simulink model "LimKyuBum_20101447_5"  (R2017a)
settings: Solver=VariableStepAuto  StartTime=0.0  StopTime=10.0  RelTol=1e-3
settings Model: Creator=508-104  LastModifiedBy=508-104

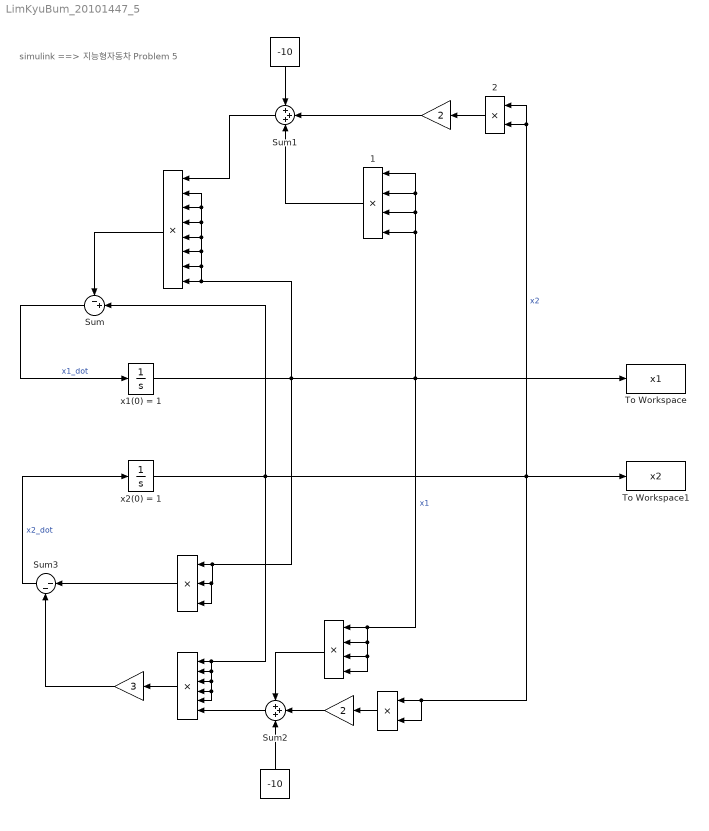
== system LimKyuBum_20101447_5 ==
  note: simulink ==> 지능형자동차 Problem 5
  " " : Product  Inputs=8
  "  " : Product  Inputs=3
  "   " : Product  Inputs=6
  "    " : Product  Inputs=4
  "     " : Product
  "      " : Gain  Gain=2
  "       " : Constant  Value=-10
  "        " : Gain  Gain=3
  "         " : Gain  Gain=2
  "          " : Constant  Value=-10
  " 1" : Product  Inputs=4
  " 2" : Product
  Sum : Sum  Inputs=-+|
  Sum1 : Sum  Inputs=+++
  Sum2 : Sum  Inputs=+++
  Sum3 : Sum  Inputs=|--
  To Workspace : ToWorkspace  VariableName=x1  SaveFormat=Timeseries  SampleTime=-1
  To Workspace1 : ToWorkspace  VariableName=x2  SaveFormat=Timeseries  SampleTime=-1
  x1(0) = 1 : Integrator  InitialCondition=1
  x2(0) = 1 : Integrator  InitialCondition=1
  wires:
  x1(0) = 1/1 -> "  "/3, "  "/2, "  "/1, " "/5, " "/2, " "/3, " "/4, " "/6, " "/7, " "/8, To Workspace/1, "    "/4, "    "/3, "    "/2, "    "/1, " 1"/3, " 1"/2, " 1"/1, " 1"/4  "x1"
  Sum/1 -> x1(0) = 1/1  "x1_dot"
  x2(0) = 1/1 -> "   "/5, "   "/4, "   "/3, "   "/2, "   "/1, To Workspace1/1, "     "/2, "     "/1, " 2"/1, " 2"/2, Sum/2  "x2"
  Sum3/1 -> x2(0) = 1/1  "x2_dot"
  " 1"/1 -> Sum1/3
  Sum1/1 -> " "/1
  " 2"/1 -> "         "/1
  "          "/1 -> Sum1/1
  "         "/1 -> Sum1/2
  " "/1 -> Sum/1
  "   "/1 -> "        "/1
  Sum2/1 -> "   "/6
  "    "/1 -> Sum2/1
  "     "/1 -> "      "/1
  "      "/1 -> Sum2/2
  "       "/1 -> Sum2/3
  "  "/1 -> Sum3/1
  "        "/1 -> Sum3/2
